simulink model "myPID"  (R2017b)
settings: Solver=VariableStepAuto  StartTime=0.0  StopTime=10.0  RelTol=1e-3
undefined symbols (not defined in the file): b, c, D, I, N, P
settings Model: Creator=apelttom  LastModifiedBy=apelttom

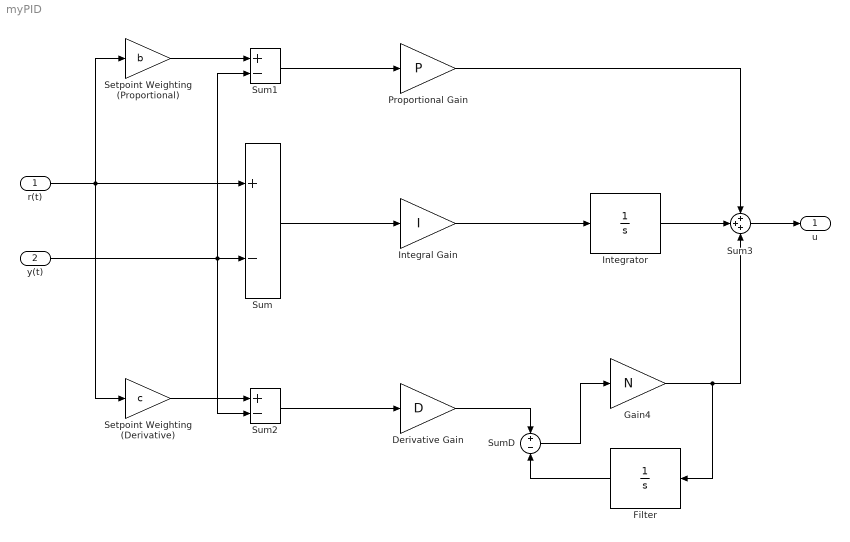
== system myPID ==
  r(t) : Inport
  y(t) : Inport  Port=2
  Derivative Gain : Gain  Gain=D
  Filter : Integrator
  Gain4 : Gain  Gain=N
  Integral Gain : Gain  Gain=I
  Integrator : Integrator  ZeroCross=off
  Proportional Gain : Gain  Gain=P
  Setpoint Weighting (Derivative) : Gain  Gain=c
  Setpoint Weighting (Proportional) : Gain  Gain=b
  Sum : Sum  Inputs=+-
  Sum1 : Sum  Inputs=+-
  Sum2 : Sum  Inputs=+-
  Sum3 : Sum  Inputs=+++
  SumD : Sum  Inputs=+-
  u : Outport
  wires:
  r(t)/1 -> Setpoint Weighting (Derivative)/1, Setpoint Weighting (Proportional)/1, Sum/1
  y(t)/1 -> Sum2/2, Sum1/2, Sum/2
  Setpoint Weighting (Derivative)/1 -> Sum2/1
  Setpoint Weighting (Proportional)/1 -> Sum1/1
  Sum1/1 -> Proportional Gain/1
  Sum/1 -> Integral Gain/1
  Integral Gain/1 -> Integrator/1
  Sum2/1 -> Derivative Gain/1
  Derivative Gain/1 -> SumD/1
  SumD/1 -> Gain4/1
  Filter/1 -> SumD/2
  Gain4/1 -> Filter/1, Sum3/3
  Integrator/1 -> Sum3/2
  Proportional Gain/1 -> Sum3/1
  Sum3/1 -> u/1
